simulink model "lab6"  (R2012b)
settings: Solver=ode45  StartTime=0.0  StopTime=720  RelTol=1e-3
undefined symbols (not defined in the file): des, gcbh
settings Model: Creator=gick  LastModifiedBy=gick

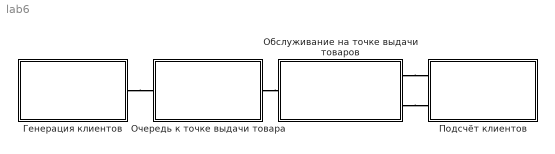
== system lab6 ==
  Генерация клиентов : Subsystem
  Обслуживание на точке выдачи товаров : Subsystem
  Очередь к точке выдачи товара : Subsystem
  Подсчёт клиентов : Subsystem
  connections:
  Генерация клиентов/RConn1 -- Очередь к точке выдачи товара/LConn1
  Очередь к точке выдачи товара/RConn1 -- Обслуживание на точке выдачи товаров/LConn1
  Обслуживание на точке выдачи товаров/RConn1 -- Подсчёт клиентов/LConn1
  Обслуживание на точке выдачи товаров/RConn2 -- Подсчёт клиентов/LConn2

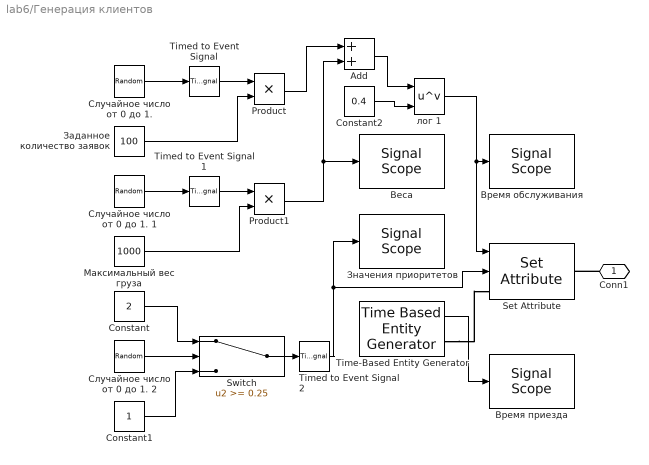
== system lab6/Генерация клиентов ==
  Add : Sum
  Constant : Constant  Value=2
  Constant1 : Constant
  Constant2 : Constant  Value=0.4
  Product : Product  RndMeth=Zero
  Product1 : Product  RndMeth=Zero
  Set Attribute : SetAttribute  AttributeName=ServTime|Priority|In  AttributeFrom=Signal port|Signal port|Dialog  AttributeValue=1|1|1  AttributeTreatAsVector=1|1|1  EvaluatedAttributeValue={ []; []; 1 }
      settings: InputPortMap=u0,u1
  Switch : Switch  Threshold=0.25
  Time-Based Entity Generator : TimeBasedEntityGenerator  Distribution=Exponential  InitialSeed=12  Mean=15  PriorityEntityGeneration=500  StatAverageIntergenerationTime=on
      settings: OutputPortMap=o2
  Timed to Event Signal : TimedToEventSignal
  Timed to Event Signal 1 : TimedToEventSignal
  Timed to Event Signal 2 : TimedToEventSignal
  Веса : SignalScope  LoadFcn=des.scope.CallbackSupport('seLoadFcn',gcbh)  StartFcn=des.scope.CallbackSupport('seStartFcn',gcbh)  StopFcn=des.scope.CallbackSupport('seStopFcn',gcbh)
      settings: CopyFcn=des.scope.CallbackSupport('seCopyFcn',gcbh)  DeleteFcn=des.scope.CallbackSupport('seDeleteFcn',gcbh)  PreSaveFcn=des.scope.CallbackSupport('sePreSaveFcn',gcbh)  NameChangeFcn=des.scope.CallbackSupport('seNameChangeFcn',gcbh)  OpenFcn=des.scope.CallbackSupport('seOpenFcn',gcbh)
  Время обслуживания : SignalScope  LoadFcn=des.scope.CallbackSupport('seLoadFcn',gcbh)  StartFcn=des.scope.CallbackSupport('seStartFcn',gcbh)  StopFcn=des.scope.CallbackSupport('seStopFcn',gcbh)  XMax=640
      settings: CopyFcn=des.scope.CallbackSupport('seCopyFcn',gcbh)  DeleteFcn=des.scope.CallbackSupport('seDeleteFcn',gcbh)  PreSaveFcn=des.scope.CallbackSupport('sePreSaveFcn',gcbh)  NameChangeFcn=des.scope.CallbackSupport('seNameChangeFcn',gcbh)  OpenFcn=des.scope.CallbackSupport('seOpenFcn',gcbh)  YMax=20
  Время приезда : SignalScope  LoadFcn=des.scope.CallbackSupport('seLoadFcn',gcbh)  StartFcn=des.scope.CallbackSupport('seStartFcn',gcbh)  StopFcn=des.scope.CallbackSupport('seStopFcn',gcbh)  XMax=640  ShowCountPlotted=on
      settings: CopyFcn=des.scope.CallbackSupport('seCopyFcn',gcbh)  DeleteFcn=des.scope.CallbackSupport('seDeleteFcn',gcbh)  PreSaveFcn=des.scope.CallbackSupport('sePreSaveFcn',gcbh)  NameChangeFcn=des.scope.CallbackSupport('seNameChangeFcn',gcbh)  OpenFcn=des.scope.CallbackSupport('seOpenFcn',gcbh)  YMax=20
  Заданное количество заявок : Constant  Value=100
  Значения приоритетов : SignalScope  LoadFcn=des.scope.CallbackSupport('seLoadFcn',gcbh)  StartFcn=des.scope.CallbackSupport('seStartFcn',gcbh)  StopFcn=des.scope.CallbackSupport('seStopFcn',gcbh)
      settings: CopyFcn=des.scope.CallbackSupport('seCopyFcn',gcbh)  DeleteFcn=des.scope.CallbackSupport('seDeleteFcn',gcbh)  PreSaveFcn=des.scope.CallbackSupport('sePreSaveFcn',gcbh)  NameChangeFcn=des.scope.CallbackSupport('seNameChangeFcn',gcbh)  OpenFcn=des.scope.CallbackSupport('seOpenFcn',gcbh)
  Максимальный вес груза : Constant  Value=1000
  Случайное число от 0 до 1. : UniformRandomNumber  Minimum=0  Seed=12  SampleTime=0.1
  "Случайное число от 0 до 1. 1 " : UniformRandomNumber  Minimum=0  Seed=12  SampleTime=0.1
  Случайное число от 0 до 1. 2 : UniformRandomNumber  Minimum=0  Seed=12  SampleTime=0.1
  лог 1 : Math  Operator=pow  SaturateOnIntegerOverflow=on
  Conn1 : PMIOPort  Port=1  Side=Right
  wires:
  Случайное число от 0 до 1./1 -> Timed to Event Signal/1
  Заданное количество заявок/1 -> Product/2
  Timed to Event Signal/1 -> Product/1
  Product/1 -> Add/1
  "Случайное число от 0 до 1. 1 "/1 -> Timed to Event Signal 1/1
  Максимальный вес груза/1 -> Product1/2
  Product1/1 -> Add/2, Веса/1
  Add/1 -> лог 1/1
  лог 1/1 -> Время обслуживания/1, Set Attribute/1
  Случайное число от 0 до 1. 2/1 -> Switch/2
  Constant/1 -> Switch/1
  Constant1/1 -> Switch/3
  Timed to Event Signal 1/1 -> Product1/1
  Switch/1 -> Timed to Event Signal 2/1
  Timed to Event Signal 2/1 -> Значения приоритетов/1, Set Attribute/2
  Time-Based Entity Generator/1 -> Время приезда/1
  Constant2/1 -> лог 1/2
  connections:
  Time-Based Entity Generator/RConn1 -- Set Attribute/LConn1
  Conn1/RConn1 -- Set Attribute/RConn1

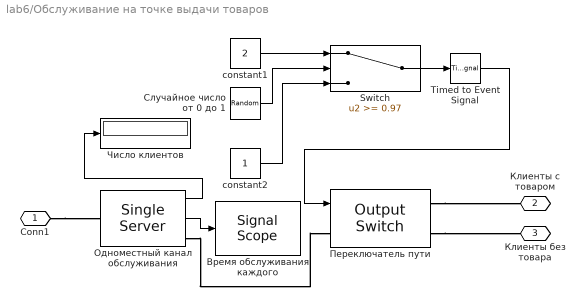
== system lab6/Обслуживание на точке выдачи товаров ==
  Switch : Switch  Threshold=0.97
  Timed to Event Signal : TimedToEventSignal
  constant1 : Constant  Value=2
  constant2 : Constant
  Время обслуживания каждого : SignalScope  LoadFcn=des.scope.CallbackSupport('seLoadFcn',gcbh)  StartFcn=des.scope.CallbackSupport('seStartFcn',gcbh)  StopFcn=des.scope.CallbackSupport('seStopFcn',gcbh)  XMax=640  ShowCountPlotted=on
      settings: CopyFcn=des.scope.CallbackSupport('seCopyFcn',gcbh)  DeleteFcn=des.scope.CallbackSupport('seDeleteFcn',gcbh)  PreSaveFcn=des.scope.CallbackSupport('sePreSaveFcn',gcbh)  NameChangeFcn=des.scope.CallbackSupport('seNameChangeFcn',gcbh)  OpenFcn=des.scope.CallbackSupport('seOpenFcn',gcbh)  YMax=20
  Одноместный канал обслуживания : SingleServer  ServiceTimeFrom=Attribute  AttributeName=ServTime  StatNumberDeparted=on  StatAverageWait=on
      settings: OutputPortMap=o0,o4
  "Переключатель пути " : OutputSwitch  NumberOutputPorts=2  SwitchingCriterion=From signal port p
  Случайное число от 0 до 1 : UniformRandomNumber  Minimum=0  Seed=12  SampleTime=0.1
  Число клиентов : Display
  Conn1 : PMIOPort  Port=1  Side=Left
  Клиенты с товаром : PMIOPort  Port=2  Side=Right
  Клиенты без товара : PMIOPort  Port=3  Side=Right
  wires:
  constant1/1 -> Switch/1
  constant2/1 -> Switch/3
  Случайное число от 0 до 1/1 -> Switch/2
  Switch/1 -> Timed to Event Signal/1
  Timed to Event Signal/1 -> "Переключатель пути "/1
  Одноместный канал обслуживания/1 -> Число клиентов/1
  Одноместный канал обслуживания/2 -> Время обслуживания каждого/1
  connections:
  "Переключатель пути "/RConn1 -- Клиенты с товаром/RConn1
  Одноместный канал обслуживания/RConn1 -- "Переключатель пути "/LConn1
  Conn1/RConn1 -- Одноместный канал обслуживания/LConn1
  "Переключатель пути "/RConn2 -- Клиенты без товара/RConn1

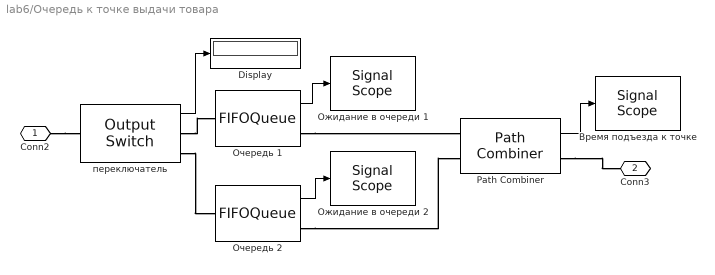
== system lab6/Очередь к точке выдачи товара ==
  Display : Display
  Path Combiner : PathCombiner  NumberInputPorts=2  StatNumberDeparted=on
  Время подъезда к точке : SignalScope  LoadFcn=des.scope.CallbackSupport('seLoadFcn',gcbh)  StartFcn=des.scope.CallbackSupport('seStartFcn',gcbh)  StopFcn=des.scope.CallbackSupport('seStopFcn',gcbh)  ShowCountPlotted=on
      settings: CopyFcn=des.scope.CallbackSupport('seCopyFcn',gcbh)  DeleteFcn=des.scope.CallbackSupport('seDeleteFcn',gcbh)  PreSaveFcn=des.scope.CallbackSupport('sePreSaveFcn',gcbh)  NameChangeFcn=des.scope.CallbackSupport('seNameChangeFcn',gcbh)  OpenFcn=des.scope.CallbackSupport('seOpenFcn',gcbh)
  Ожидание в очереди 1 : SignalScope  LoadFcn=des.scope.CallbackSupport('seLoadFcn',gcbh)  StartFcn=des.scope.CallbackSupport('seStartFcn',gcbh)  StopFcn=des.scope.CallbackSupport('seStopFcn',gcbh)  ShowCountPlotted=on
      settings: CopyFcn=des.scope.CallbackSupport('seCopyFcn',gcbh)  DeleteFcn=des.scope.CallbackSupport('seDeleteFcn',gcbh)  PreSaveFcn=des.scope.CallbackSupport('sePreSaveFcn',gcbh)  NameChangeFcn=des.scope.CallbackSupport('seNameChangeFcn',gcbh)  OpenFcn=des.scope.CallbackSupport('seOpenFcn',gcbh)
  Ожидание в очереди 2 : SignalScope  LoadFcn=des.scope.CallbackSupport('seLoadFcn',gcbh)  StartFcn=des.scope.CallbackSupport('seStartFcn',gcbh)  StopFcn=des.scope.CallbackSupport('seStopFcn',gcbh)  ShowCountPlotted=on
      settings: CopyFcn=des.scope.CallbackSupport('seCopyFcn',gcbh)  DeleteFcn=des.scope.CallbackSupport('seDeleteFcn',gcbh)  PreSaveFcn=des.scope.CallbackSupport('sePreSaveFcn',gcbh)  NameChangeFcn=des.scope.CallbackSupport('seNameChangeFcn',gcbh)  OpenFcn=des.scope.CallbackSupport('seOpenFcn',gcbh)
  Очередь 1 : FIFOQueue  Capacity=10  StatAverageWait=on
      settings: OutputPortMap=o2
  "Очередь 2 " : FIFOQueue  Capacity=10  StatAverageWait=on
      settings: OutputPortMap=o2
  "переключатель " : OutputSwitch  NumberOutputPorts=2  SwitchingCriterion=From attribute  AttributeName=Priority  StatNumberDeparted=on
  Conn2 : PMIOPort  Port=1  Side=Left
  Conn3 : PMIOPort  Port=2  Side=Right
  wires:
  Path Combiner/1 -> Время подъезда к точке/1
  "переключатель "/1 -> Display/1
  Очередь 1/1 -> Ожидание в очереди 1/1
  "Очередь 2 "/1 -> Ожидание в очереди 2/1
  connections:
  "переключатель "/RConn2 -- "Очередь 2 "/LConn1
  Conn2/RConn1 -- "переключатель "/LConn1
  Path Combiner/RConn1 -- Conn3/RConn1
  "переключатель "/RConn1 -- Очередь 1/LConn1
  Очередь 1/RConn1 -- Path Combiner/LConn1
  "Очередь 2 "/RConn1 -- Path Combiner/LConn2

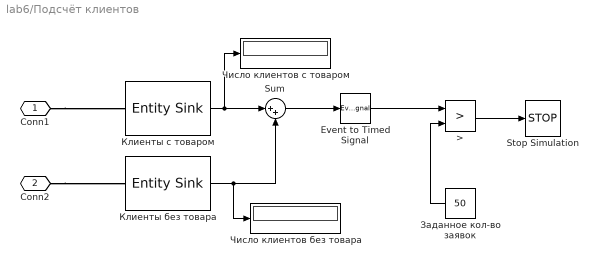
== system lab6/Подсчёт клиентов ==
  > : RelationalOperator  Operator=>  OutDataTypeStr=boolean
  Event to Timed Signal : EventToTimedSignal
  Stop Simulation : Stop
  Sum : Sum  Inputs=|++
  Заданное кол-во заявок : Constant  Value=50
  Клиенты без товара : EntitySink  StatNumberArrived=on
  Клиенты с товаром : EntitySink  StatNumberArrived=on
  Число клиентов без товара : Display
  Число клиентов с товаром : Display
  Conn1 : PMIOPort  Port=1  Side=Left
  Conn2 : PMIOPort  Port=2  Side=Left
  wires:
  Клиенты с товаром/1 -> Число клиентов с товаром/1, Sum/1
  Клиенты без товара/1 -> Число клиентов без товара/1, Sum/2
  Sum/1 -> Event to Timed Signal/1
  Заданное кол-во заявок/1 -> >/2
  Event to Timed Signal/1 -> >/1
  >/1 -> Stop Simulation/1
  connections:
  Conn2/RConn1 -- Клиенты без товара/LConn1
  Conn1/RConn1 -- Клиенты с товаром/LConn1
